simulink model "SMC"  (Simulink 8.7)
settings: Solver=ode45  StartTime=0.0  StopTime=inf  MaxStep=0.02  RelTol=1e-3
values from neighbouring files (symbols this model uses):
  A = [0 1;0 -Kf/I]    [Observador_Ivan.m]
  B = [0;Conv1*Kv*L1/I]    [Observador_Ivan.m]
  C = [1 0]    [Observador_Ivan.m]
  L = PObs*Lbarra    [Observador_Ivan.m]
libraries: arduino_io_lib x5
settings Model: Creator=Administrador  LastModifiedBy=Sergio Toledo
settings DataIOCC: SignalLoggingSaveFormat=ModelDataLogs
settings OptimizationCC: ExpressionDepthLimit=2147483647  InitFltsAndDblsToZero=on
settings DebuggingCC: SolverPrmCheckMsg=warning  FcnCallInpInsideContextMsg=UseLocalSettings  StateNameClashWarn=warning
settings GRTTargetCC: CombineOutputUpdateFcns=off  GRTInterface=on

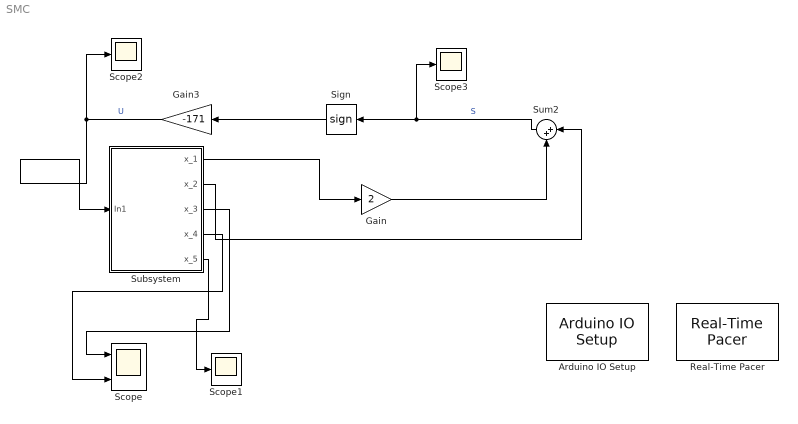
== system SMC ==
  Arduino IO Setup : arduino_io_lib/Arduino IO Setup  Priority=3  arduinoVar=Existing workspace arduino variable #1  workspaceVarName=ard  comPort=4
  Gain : Gain  Gain=2
  Gain3 : Gain  Gain=-171
  Real-Time Pacer : arduino_io_lib/Real-Time Pacer  simTimePerRealTime=1
  Scope : Scope  NumInputPorts=2
  Scope1 : Scope
  Scope2 : Scope
  Scope3 : Scope
  Sign : Signum  ZeroCross=off
  Subsystem : Subsystem
  Sum2 : Sum  Inputs=|++
  wires:
  Sum2/1 -> Scope3/1, Sign/1  "S"
  Sign/1 -> Gain3/1
  Gain3/1 -> Subsystem/1(In1), Scope2/1  "U"
  Subsystem/2(x_2) -> Sum2/1
  Gain/1 -> Sum2/2
  Subsystem/1(x_1) -> Gain/1
  Subsystem/3(x_3) -> Scope/1
  Subsystem/4(x_4) -> Scope/2
  Subsystem/5(x_5) -> Scope1/1

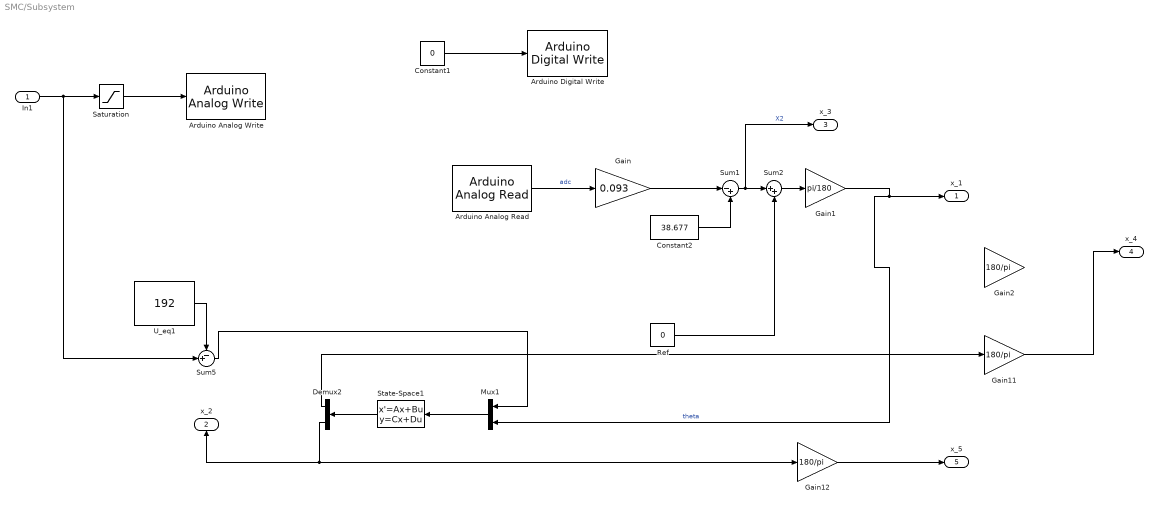
== system SMC/Subsystem ==
  In1 : Inport
  Arduino Analog Read : arduino_io_lib/Arduino Analog Read  arduinoVar=Existing workspace arduino variable #1  arduinoPin=8  T=0.1
  Arduino Analog Write : arduino_io_lib/Arduino Analog Write  arduinoVar=Existing workspace arduino variable #1  arduinoPin=3  T=0.1
  Arduino Digital Write : arduino_io_lib/Arduino Digital Write  arduinoVar=Existing workspace arduino variable #1  arduinoPin=12  T=0.1
  Constant1 : Constant  Value=0
  Constant2 : Constant  Value=38.677
  Demux2 : Demux  Outputs=2
  Gain : Gain  Gain=0.093
  Gain1 : Gain  Gain=pi/180
  Gain11 : Gain  Gain=180/pi
  Gain12 : Gain  Gain=180/pi
  Gain2 : Gain  Gain=180/pi
  Mux1 : Mux  Inputs=2
  Ref : Constant  Value=0
  Saturation : Saturate  UpperLimit=255  LowerLimit=150  ZeroCross=off
  State-Space1 : StateSpace  A=A-L*C  B=[B L]  C=eye(2)  D=zeros(2,2)  X0=[-0.65 0]
  Sum1 : Sum  Inputs=|-+
  Sum2 : Sum  Inputs=|++
  Sum5 : Sum  Inputs=-+|
  U_eq1 : Constant  Value=192
  x_1 : Outport
  x_2 : Outport  Port=2
  x_3 : Outport  Port=3
  x_4 : Outport  Port=4
  x_5 : Outport  Port=5
  wires:
  Arduino Analog Read/1 -> Gain/1  "adc"
  Constant1/1 -> Arduino Digital Write/1
  Gain/1 -> Sum1/1
  Constant2/1 -> Sum1/2
  Gain1/1 -> Mux1/2, x_1/1  "theta"
  State-Space1/1 -> Demux2/1
  Mux1/1 -> State-Space1/1
  Sum5/1 -> Mux1/1
  U_eq1/1 -> Sum5/1
  Gain12/1 -> x_5/1
  Demux2/2 -> x_2/1, Gain12/1
  Demux2/1 -> Gain11/1
  Gain11/1 -> x_4/1
  Saturation/1 -> Arduino Analog Write/1
  In1/1 -> Sum5/2, Saturation/1
  Sum1/1 -> x_3/1, Sum2/1  "X2"
  Ref/1 -> Sum2/2
  Sum2/1 -> Gain1/1
